simulink model "ControlSchemeModel"  (R2019b)
settings: Solver=VariableStepAuto  StartTime=0.0  StopTime=10.0  RelTol=1e-3
libraries: simulink x1
settings Model: Creator=marco  LastModifiedBy=marco

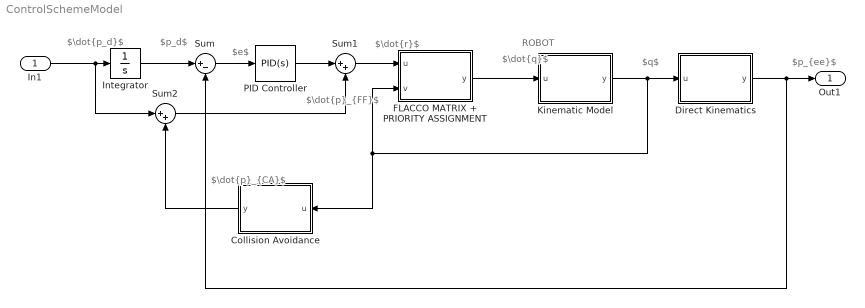
== system ControlSchemeModel ==
  note: ROBOT
  note: $e$
  note: $\dot{r}$
  note: $\dot{p}_{FF}$
  note: $\dot{p}_{CA}$
  note: $\dot{q}$
  note: $q$
  note: $p_{ee}$
  note: $p_d$
  note: $\dot{p_d}$
  In1 : Inport
  "Collision Avoidance " : MATLAB Function  TreatAsAtomicUnit=on
  Direct Kinematics : MATLAB Function  TreatAsAtomicUnit=on
  "FLACCO MATRIX + PRIORITY ASSIGNMENT " : MATLAB Function  TreatAsAtomicUnit=on
  Integrator : Integrator
  Kinematic Model : MATLAB Function  TreatAsAtomicUnit=on
  PID Controller : simulink/Continuous/PID Controller  Controller=PID  Form=Parallel  TimeDomain=Continuous-time  SampleTime=-1  IntegratorMethod=Forward Euler  FilterMethod=Forward Euler  ControllerParametersSource=internal  P=1  I=1  D=0  UseFilter=on  N=100  TunerSelectOption=Transfer Function Based (PID Tuner App)  InitialConditionSource=internal  InitialConditionForIntegrator=0  InitialConditionForFilter=0  DifferentiatorICPrevScaledInput=0  ExternalReset=none  TrackingMode=off  Kt=1  LimitOutput=off  UpperSaturationLimit=inf  LowerSaturationLimit=-inf  LinearizeAsGain=on  AntiWindupMode=none  Kb=1  POutMin=[]  POutMax=[]  IOutMin=[]  IOutMax=[]  DOutMin=[]  DOutMax=[]  NOutMin=[]  NOutMax=[]  SumOutMin=[]  SumOutMax=[]  SaturationOutMin=[]  SaturationOutMax=[]  PParamMin=[]  PParamMax=[]  IParamMin=[]  IParamMax=[]  DParamMin=[]  DParamMax=[]  NParamMin=[]  NParamMax=[]  KbParamMin=[]  KbParamMax=[]  KtParamMin=[]  KtParamMax=[]  KbOutMin=[]  KbOutMax=[]  KtOutMin=[]  KtOutMax=[]  IntegratorOutMin=[]  IntegratorOutMax=[]  FilterOutMin=[]  FilterOutMax=[]  SumI1OutMin=[]  SumI1OutMax=[]  SumI2OutMin=[]  SumI2OutMax=[]  SumI3OutMin=[]  SumI3OutMax=[]  SumI4OutMin=[]  SumI4OutMax=[]  SumDOutMin=[]  SumDOutMax=[]  DifferentiatorOutMin=[]  DifferentiatorOutMax=[]  FilterDiffOutCoefMin=[]  FilterDiffOutCoefMax=[]  ReciprocalOutMin=[]  ReciprocalOutMax=[]  SumDenOutMin=[]  SumDenOutMax=[]  SumNumOutMin=[]  SumNumOutMax=[]  DivideOutMin=[]  DivideOutMax=[]  IntegratorContinuousStateAttributes=''  IntegratorStateMustResolveToSignalObject=off  IntegratorRTWStateStorageClass=Auto  FilterContinuousStateAttributes=''  FilterStateMustResolveToSignalObject=off  FilterRTWStateStorageClass=Auto  ParallelPVariant=InternalParameters  IdealPVariant=Disabled  IVariant=InternalParameters  DVariant=InternalParameters  IntegratorVariant=Continuous  SatVariant=Disabled  AWVariant=Passthrough  PCopyVariant=Disabled  TRVariant=Disabled  FdbkBlocksVariant=Forward  IdealPFdbkVariant=Disabled  SatFdbkVariant=Disabled  DerivativeFilterVariant=ContFilter  NVariant=InternalParameters  NCopyVariant=Disabled  FilterICVariant=InternalICsFilter  IntegratorICVariant=InternalICs  ExternalResetVariant=Disabled  TRSumVariant=Passthrough  SumFdbkVariant=Disabled  SumVariant=Sum_PID
  Sum : Sum  Inputs=|+-
  Sum1 : Sum  Inputs=|++
  Sum2 : Sum  Inputs=|++
  Out1 : Outport
  wires:
  Integrator/1 -> Sum/1
  Sum/1 -> PID Controller/1
  In1/1 -> Sum2/1, Integrator/1
  PID Controller/1 -> Sum1/1
  Sum1/1 -> "FLACCO MATRIX + PRIORITY ASSIGNMENT "/1(u)
  "FLACCO MATRIX + PRIORITY ASSIGNMENT "/1(y) -> Kinematic Model/1(u)
  Kinematic Model/1(y) -> "Collision Avoidance "/1(u), "FLACCO MATRIX + PRIORITY ASSIGNMENT "/2(v), Direct Kinematics/1(u)
  Direct Kinematics/1(y) -> Sum/2, Out1/1
  Sum2/1 -> Sum1/2
  "Collision Avoidance "/1(y) -> Sum2/2

== matlab function ControlSchemeModel/Kinematic Model ==
  data: u input; y output
function y = fcn(u)

y = u;

== matlab function ControlSchemeModel/FLACCO MATRIX + PRIORITY ASSIGNMENT  ==
  data: u input; y output; v input
function y = fcn(u,v)

y = u;
end

== matlab function ControlSchemeModel/Direct Kinematics ==
  data: u input; y output
function y = fcn(u)

y = u;

== matlab function ControlSchemeModel/Collision Avoidance  ==
  data: y output; u input
function y = fcn(u)

y = 1;
end
